simulink model "cacc_consensus_test_error"  (R2022b)
settings: Solver=VariableStepAuto  StartTime=0.0  StopTime=60  RelTol=1e-3
values from neighbouring files (symbols this model uses):
  A = [0 1 0; 0 0 1; 0 0 -1/tau]    [cacc_consensus_main.m]    (also in dyn_graph.m; dyn_graph_10.m; dyn_graph_10_disturb.m; fixed_graph.m)
  B = [0 0 1/tau]'    [cacc_consensus_main.m]    (also in dyn_graph.m; dyn_graph_10.m; dyn_graph_10_disturb.m; fixed_graph.m)
  C = diag([1 1 1])    [cacc_consensus_main.m]    (also in dyn_graph.m; dyn_graph_10.m; dyn_graph_10_disturb.m; fixed_graph.m)
  D = [0 0 0]'    [cacc_consensus_main.m]    (also in dyn_graph.m; dyn_graph_10.m; dyn_graph_10_disturb.m; fixed_graph.m)
  K_cacc = K_lqr    [cacc_consensus_main.m]    (also in dyn_graph.m = -K_lmi; fixed_graph.m = -K_lmi; fixed_graph_lpv.m = -K_lmi)
libraries: cstblocks x4, simulink x1
settings Model: Creator=phatdo  LastModifiedBy=phatdo
settings DataIOCC: ReturnWorkspaceOutputs=off

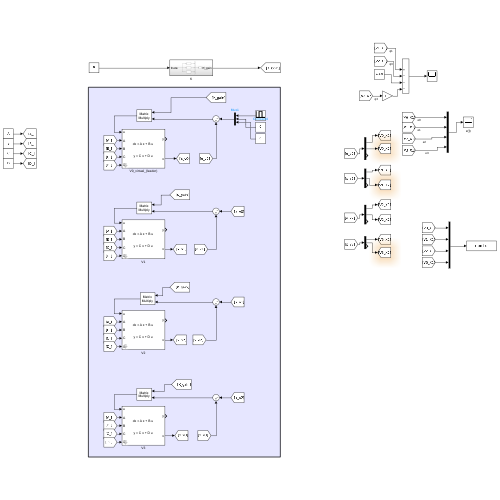
[thumbnail: Simulink's stored preview of the top-level diagram]
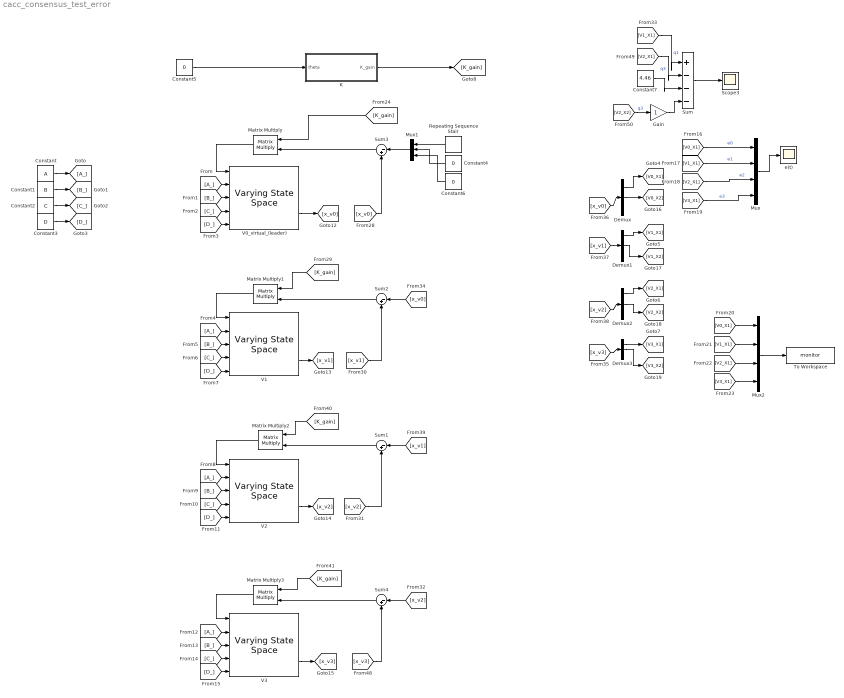
== system cacc_consensus_test_error ==
  Constant : Constant  Value=A
  Constant1 : Constant  Value=B
  Constant2 : Constant  Value=C
  Constant3 : Constant  Value=D
  Constant4 : Constant  Value=0
  Constant5 : Constant  Value=0
  Constant6 : Constant  Value=0
  Constant7 : Constant  Value=4.46
  Demux{,1..3} (4 alike) : Demux  Outputs=3
  Gain : Gain
  K : Subsystem
  Matrix Multiply{,1..3} (4 alike) : Product  Multiplication=Matrix(*)
  Mux : Mux
  Mux1 : Mux  Inputs=3
  Mux2 : Mux
  Repeating Sequence Stair : simulink/Sources/Repeating Sequence Stair  OutValues=[0 5 0]  tsamp=20  OutMin=[]  OutMax=[]  OutDataTypeStr=double  OutputDataTypeScalingMode=double  OutDataType=fixdt(0,8)  ConRadixGroup=Best Precision: Vector-wise  OutScaling=2^-12
  Scope3 : Scope
  Sum : Sum  Inputs=|+---
  Sum{1..4} (4 alike) : Sum  Inputs=|-+
  To Workspace : ToWorkspace  VariableName=monitor  SaveFormat=Timeseries  SampleTime=-1
  V0_virtual_(leader) : cstblocks/Linear Parameter Varying/Varying State Space  x0=[0;0;0]  xNames=''  OutputX=on  OutputDX=off
  V1 : cstblocks/Linear Parameter Varying/Varying State Space  x0=[0.7;0;0]  xNames=''  OutputX=on  OutputDX=off
  V2 : cstblocks/Linear Parameter Varying/Varying State Space  x0=[0.4;0;0]  xNames=''  OutputX=on  OutputDX=off
  V3 : cstblocks/Linear Parameter Varying/Varying State Space  x0=[-1 ;0 ; 0]  xNames=''  OutputX=on  OutputDX=off
  e(t) : Scope
  wires:
  Sum3/1 -> Matrix Multiply/2
  Sum2/1 -> Matrix Multiply1/2
  Sum1/1 -> Matrix Multiply2/2
  Constant2/1 -> [C_]
  Constant/1 -> [A_]
  Constant3/1 -> [D_]
  Constant1/1 -> [B_]
  [B_] -> V0_virtual_(leader)/3
  [A_] -> V0_virtual_(leader)/2
  [C_] -> V0_virtual_(leader)/4
  [D_] -> V0_virtual_(leader)/5
  [D_] -> V1/5
  [A_] -> V2/2
  [A_] -> V3/2
  [A_] -> V1/2
  [B_] -> V1/3
  [C_] -> V1/4
  [B_] -> V2/3
  [C_] -> V2/4
  [D_] -> V2/5
  [B_] -> V3/3
  [C_] -> V3/4
  [D_] -> V3/5
  [V2_X1] -> Mux/3  "e2"
  [V3_X1] -> Mux/4  "e3"
  Mux/1 -> e(t)/1
  [V1_X1] -> Mux/2  "e1"
  [V0_X1] -> Mux/1  "e0"
  Constant5/1 -> K/1(theta)
  [V1_X1] -> Mux2/2
  [V0_X1] -> Mux2/1
  [V3_X1] -> Mux2/4
  Mux2/1 -> To Workspace/1
  [V2_X1] -> Mux2/3
  K/1(K_gain) -> [K_gain]
  [K_gain] -> Matrix Multiply/1
  Matrix Multiply/1 -> V0_virtual_(leader)/1
  V0_virtual_(leader)/2 -> [x_v0]
  Matrix Multiply1/1 -> V1/1
  [K_gain] -> Matrix Multiply1/1
  V1/2 -> [x_v1]
  [x_v0] -> Sum3/2
  [x_v1] -> Sum2/2
  Matrix Multiply2/1 -> V2/1
  V2/2 -> [x_v2]
  [x_v2] -> Sum1/2
  V3/2 -> [x_v3]
  Mux1/1 -> Sum3/1
  [x_v0] -> Sum2/1
  [x_v1] -> Sum1/1
  [x_v0] -> Demux/1
  [x_v1] -> Demux1/1
  [x_v2] -> Demux2/1
  [x_v3] -> Demux3/1
  [K_gain] -> Matrix Multiply2/1
  Matrix Multiply3/1 -> V3/1
  [K_gain] -> Matrix Multiply3/1
  Demux/1 -> [V0_X1]
  Demux1/1 -> [V1_X1]
  Demux2/1 -> [V2_X1]
  Demux3/1 -> [V3_X1]
  Demux/2 -> [V0_X2]
  Demux1/2 -> [V1_X2]
  Demux2/2 -> [V2_X2]
  Demux3/2 -> [V3_X2]
  [x_v3] -> Sum4/2
  Sum4/1 -> Matrix Multiply3/2
  [x_v2] -> Sum4/1
  [V1_X1] -> Sum/1  "q1"
  [V2_X1] -> Sum/2  "q3"
  Constant7/1 -> Sum/3
  Gain/1 -> Sum/4
  Sum/1 -> Scope3/1
  [V2_X2] -> Gain/1  "q3"
  Repeating Sequence Stair/1 -> Mux1/1
  Constant4/1 -> Mux1/2
  Constant6/1 -> Mux1/3

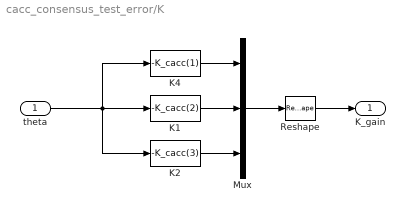
== system cacc_consensus_test_error/K ==
  theta : Inport
  K1 : Fcn  Expr=-K_cacc(2)
  K2 : Fcn  Expr=-K_cacc(3)
  K4 : Fcn  Expr=-K_cacc(1)
  Mux : Mux  Inputs=3
  Reshape : Reshape  OutputDimensionality=Customize  OutputDimensions=[1,3]
  K_gain : Outport
  wires:
  Mux/1 -> Reshape/1
  Reshape/1 -> K_gain/1
  K4/1 -> Mux/1
  K1/1 -> Mux/2
  K2/1 -> Mux/3
  theta/1 -> K2/1, K1/1, K4/1
